simulink model "questao3Miguel"  (Simulink 8.7)
settings: Solver=ode45  StartTime=0.0  StopTime=40  MaxStep=0.01  RelTol=1e-3
values from neighbouring files (symbols this model uses):
  A = [0 1  0              0 ... (first row only)    [MatLab4p.m]    (also in MatLab5p.m = [     0        1       0        0; MatLab6p_solucao4.m = [     0        1       0        0; MatLab7p.m = [0 1; -5*sqrt(2) -1]; pplane8.m = [)
  Am = blkdiag(M,M)    [MatLab5p.m]    (also in MatLab6p_solucao4.m; questao2Miguel.m = blkdiag(M); questao2MiguelFinal.m = blkdiag(M))
  B = [0; 1/M; 0; -1/(M*L)]    [MatLab4p.m]    (also in MatLab5p.m = [ 0    0; MatLab6p_solucao4.m = [ 0    0; MatLab7p.m = [0 ; 10]; pplane8.m = real(A))
  Bm = blkdiag(N,N)    [MatLab5p.m]    (also in MatLab6p_solucao4.m; questao2Miguel.m = blkdiag(N); questao2MiguelFinal.m = blkdiag(N))
  C = [1 0 0 0]    [MatLab4p.m]    (also in MatLab5p.m = [1 0 0 0; MatLab6p_solucao4.m = [1 0 0 0; MatLab7p.m = [1 0]; pplane8.m = imag(A))
  Dsim = zeros(4,1)    [MatLab4p.m]    (also in MatLab5p.m = zeros(4,2); MatLab6p_solucao4.m = zeros(4,2); questao2Miguel.m; questao2MiguelFinal.m)
  g = 9.81    [MatLab4p.m]    (also in PenduloInvertidoNLinear.m; questao2Miguel.m; questao2MiguelFinal.m)
  K = place(A,B,[-3 -3.05 -3.1 -3.15])    [MatLab4p.m]    (also in MatLab5p.m = Ka(:,1:4); MatLab6p_solucao4.m = Ka(:,1:4); MatLab7p.m = place(A,B,[-4 -4.05]); pplane8.m = kk +2*(jj-1))
  Km = Ka(:,5:10)    [MatLab5p.m]    (also in MatLab6p_solucao4.m = Ka(:,5:12); MatLab7p.m = Ka(1,3); questao2Miguel.m = Ka(5); questao2MiguelFinal.m = Ka(5))
  L = (place(A',C',[-9 -9.05 -9.1 -9.15]))'    [MatLab4p.m]    (also in MatLab7p.m = [23 ; 113.9289]; PenduloInvertidoNLinear.m = 1; pplane8.m = length(t); questao2Miguel.m = 1)
  Lobs = H'    [MatLab6p_solucao4.m]    (also in questao2Miguel.m; questao2MiguelFinal.m)
  m = 0.5    [MatLab4p.m]    (also in PenduloInvertidoNLinear.m; questao2Miguel.m; questao2MiguelFinal.m)
  Mcar = 1    [questao2MiguelFinal.m]
  x0 = [0 0 pi/4 0]    [MatLab4p.m]    (also in MatLab5p.m = [1 0.5 1 0.1]; MatLab6p_solucao4.m = [0 0 0 0]; MatLab7p.m = [0 ; 0]; questao2Miguel.m = [0 0.01 0.3 0])
  x0obs = [0 0 0 0]    [MatLab4p.m]    (also in MatLab6p_solucao4.m; MatLab7p.m = [0 ; 0]; questao2Miguel.m; questao2MiguelFinal.m)
  xe = [0 0 pi 0]    [questao2MiguelFinal.m]
settings Model: Creator=hector  LastModifiedBy=Deinis-UFSC
settings DebuggingCC: UnderspecifiedInitializationDetection=Simplified  MergeDetectMultiDrivingBlocksExec=error  SolverPrmCheckMsg=warning
settings ConfigComp: CovSFcnEnable=off

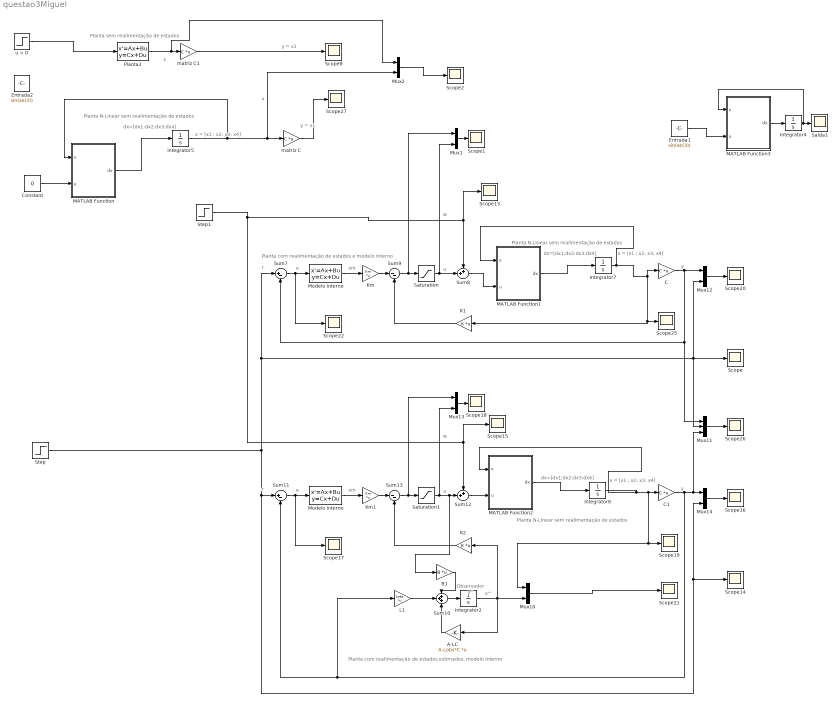
== system questao3Miguel ==
  note: Planta com realimentação de estados estimados, modelo interno
  note: Planta com realimentação de estados e modelo interno
  note: w
  note: u
  note: xm
  note: e
  note: r
  note: y
  note: w
  note: u
  note: xm
  note: e
  note: r
  note: y
  note: Observador
  note: x^
  note: x^
  note: Planta N-Linear sem realimentação de estados
  note: x
  note: y = x1
  note: dx=[dx1;dx2;dx3;dx4]
  note: x = [x1 ; x2; x3; x4]
  note: Planta N-Linear sem realimentação de estados
  note: dx=[dx1;dx2;dx3;dx4]
  note: x = [x1 ; x2; x3; x4]
  note: Planta N-Linear sem realimentação de estados
  note: dx=[dx1;dx2;dx3;dx4]
  note: x = [x1 ; x2; x3; x4]
  note: Planta sem realimentação de estados
  note: x
  note: y = x1
  A-LC : Gain  Gain=A-Lobs*C  Multiplication=Matrix(K*u)
  B1 : Gain  Gain=B  Multiplication=Matrix(K*u)
  C : Gain  Gain=C  Multiplication=Matrix(K*u)
  C1 : Gain  Gain=C  Multiplication=Matrix(K*u)
  Constant : Constant  Value=0
  Entrada1 : Constant  Value=sin(xe(3))
  Entrada2 : Constant  Value=sin(xe(3))
  Integrator2 : Integrator  InitialCondition=x0obs
  Integrator4 : Integrator  InitialCondition=xe
  Integrator5 : Integrator  InitialCondition=x0
  Integrator7 : Integrator  InitialCondition=x0
  Integrator8 : Integrator  InitialCondition=x0
  K1 : Gain  Gain=K  Multiplication=Matrix(K*u)
  K2 : Gain  Gain=K  Multiplication=Matrix(K*u)
  Km : Gain  Gain=Km  Multiplication=Matrix(K*u)
  Km1 : Gain  Gain=Km  Multiplication=Matrix(K*u)
  L1 : Gain  Gain=Lobs  Multiplication=Matrix(K*u)
  MATLAB Function : MATLAB Function  TreatAsAtomicUnit=on
  MATLAB Function1 : MATLAB Function  TreatAsAtomicUnit=on
  MATLAB Function2 : MATLAB Function  TreatAsAtomicUnit=on
  MATLAB Function3 : MATLAB Function  TreatAsAtomicUnit=on
  Modelo Interno : StateSpace  A=Am  B=Bm  D=0  X0=0
  Modelo interno : StateSpace  A=Am  B=Bm  D=0  X0=0
  Mux{1..2,10,12..14} (6 alike) : Mux  Inputs=2
  Mux11 : Mux  Inputs=3
  Planta2 : StateSpace  A=A  B=B  C=eye(4)  D=Dsim  X0=x0
  Saida1 : Scope
  Saturation : Saturate  UpperLimit=50  LowerLimit=-50
  Saturation1 : Saturate  UpperLimit=50  LowerLimit=-50
  Scope{,1..2,8,13..22,25..27} (17 alike) : Scope
  Step : Step  Time=5  SampleTime=0
  Step1 : Step  Time=15  After=0.5  SampleTime=0
  Sum10 : Sum  Inputs=+++
  Sum11 : Sum  Inputs=|+-
  Sum12 : Sum  Inputs=++|
  Sum13 : Sum  Inputs=|--
  Sum7 : Sum  Inputs=|+-
  Sum8 : Sum  Inputs=++|
  Sum9 : Sum  Inputs=|--
  matriz C : Gain  Gain=C  Multiplication=Matrix(K*u)
  matriz C1 : Gain  Gain=C  Multiplication=Matrix(K*u)
  "u = 0 " : Step  Time=0  After=0  SampleTime=0
  wires:
  Sum7/1 -> Modelo Interno/1, Scope22/1
  Mux12/1 -> Scope20/1
  Km/1 -> Sum9/1
  Modelo Interno/1 -> Km/1
  K1/1 -> Sum9/2
  Step/1 -> Sum7/1, Mux11/2, Scope/1, Mux12/2, Sum11/1, Scope14/1, Mux14/2
  Sum11/1 -> Modelo interno/1, Scope17/1
  Step1/1 -> Sum12/1, Scope15/1, Sum8/1, Scope13/1
  Mux14/1 -> Scope16/1
  Sum13/1 -> Mux13/1, Saturation1/1
  Km1/1 -> Sum13/1
  Modelo interno/1 -> Km1/1
  K2/1 -> Sum13/2
  Sum10/1 -> Integrator2/1
  L1/1 -> Sum10/2
  A-LC/1 -> Sum10/3
  B1/1 -> Sum10/1
  Mux10/1 -> Scope21/1
  Mux11/1 -> Scope26/1
  matriz C/1 -> Scope27/1
  Mux13/1 -> Scope18/1
  Constant/1 -> MATLAB Function/2(u)
  Sum8/1 -> MATLAB Function1/2(u)
  MATLAB Function1/1(dx) -> Integrator7/1
  Sum12/1 -> MATLAB Function2/2(u)
  MATLAB Function2/1(dx) -> Integrator8/1
  C1/1 -> L1/1, Sum11/2, Mux11/3, Mux14/1
  C/1 -> Mux12/1, Sum7/2, Mux11/1
  Integrator5/1 -> MATLAB Function/1(x), Mux2/2, matriz C/1
  Integrator7/1 -> MATLAB Function1/1(x), K1/1, Scope25/1, C/1
  Saturation1/1 -> Mux13/2, B1/1, Sum12/2
  Integrator2/1 -> A-LC/1, Mux10/2, K2/1
  Integrator8/1 -> Mux10/1, Scope19/1, C1/1, MATLAB Function2/1(x)
  MATLAB Function/1(dx) -> Integrator5/1
  Sum9/1 -> Mux1/1, Saturation/1
  Mux1/1 -> Scope1/1
  Saturation/1 -> Mux1/2, Sum8/2
  MATLAB Function3/1(dx) -> Integrator4/1
  Integrator4/1 -> MATLAB Function3/1(x), Saida1/1
  Entrada1/1 -> MATLAB Function3/2(u)
  "u = 0 "/1 -> Planta2/1
  matriz C1/1 -> Scope8/1
  Planta2/1 -> Mux2/1, matriz C1/1
  Mux2/1 -> Scope2/1

== matlab function MATLAB Function1 ==
  data: x input double; u input double; dx output double; m parameter double; Mcar parameter double; L parameter double; g parameter double
function dx = fcn(x,u,m, Mcar, L, g)
%#codegen

% dx1 = x(2);
% dx2 = u - (m*g*cos(x(3))*sin(x(3))+m*L*x(4)^2*sin(x(3)))/(Mcar+m - m*cos(x(3))^2);
% dx3 = x(4);
% dx4 = (u*cos(x(3))+m*L*x(4)^2*cos(x(3))*sin(x(3))-(Mcar+m)*g*sin(x(3)))/(m*L*cos(x(3))^2 - L*(Mcar+m));

dx1 = x(2);
dx2 = (m*L*x(4)^2*sin(x(3))-m*g*sin(x(3))*cos(x(3)) + u)/((Mcar+m*sin(x(3))^2)*L);
dx3 = x(4);
dx4 = ((Mcar+m)*g*sin(x(3)) + m*L*x(4)^2*sin(x(3))*cos(x(3)) - u*cos(x(3)))/((Mcar+m*sin(x(3))^2)*L);

dx = [dx1 ; dx2 ; dx3 ; dx4];

== matlab function MATLAB Function ==
  data: x input double; u input double; dx output double; m parameter double; Mcar parameter double; L parameter double; g parameter double
function dx = fcn(x,u,m, Mcar, L, g)
%#codegen

% dx1 = x(2);
% dx2 = u - (m*g*cos(x(3))*sin(x(3))+m*L*x(4)^2*sin(x(3)))/(Mcar+m - m*cos(x(3))^2);
% dx3 = x(4);
% dx4 = (u*cos(x(3))+m*L*x(4)^2*cos(x(3))*sin(x(3))-(Mcar+m)*g*sin(x(3)))/(m*L*cos(x(3))^2 - L*(Mcar+m));

dx1 = x(2);
dx2 = (m*L*x(4)^2*sin(x(3))-m*g*sin(x(3))*cos(x(3)) + u)/((Mcar+m*sin(x(3))^2)*L);
dx3 = x(4);
dx4 = ((Mcar+m)*g*sin(x(3)) + m*L*x(4)^2*sin(x(3))*cos(x(3)) - u*cos(x(3)))/((Mcar+m*sin(x(3))^2)*L);

dx = [dx1 ; dx2 ; dx3 ; dx4];

== matlab function MATLAB Function2 ==
  data: x input double; u input double; dx output double; m parameter double; Mcar parameter double; L parameter double; g parameter double
function dx = fcn(x,u,m, Mcar, L, g)
%Miguel 

% dx1 = x(2);
% dx2 = u - (m*g*cos(x(3))*sin(x(3))+m*L*x(4)^2*sin(x(3)))/(Mcar+m - m*cos(x(3))^2);
% dx3 = x(4);
% dx4 = (u*cos(x(3))+m*L*x(4)^2*cos(x(3))*sin(x(3))-(Mcar+m)*g*sin(x(3)))/(m*L*cos(x(3))^2 - L*(Mcar+m));

dx1 = x(2);
dx2 = (m*L*x(4)^2*sin(x(3))-m*g*sin(x(3))*cos(x(3)) + u)/((Mcar+m*sin(x(3))^2)*L);
dx3 = x(4);
dx4 = ((Mcar+m)*g*sin(x(3)) + m*L*x(4)^2*sin(x(3))*cos(x(3)) - u*cos(x(3)))/((Mcar+m*sin(x(3))^2)*L);


dx = [dx1 ; dx2 ; dx3 ; dx4];

== matlab function MATLAB Function3 ==
  data: x input double; u input double; dx output double; m parameter double; Mcar parameter double; L parameter double; g parameter double
function dx = fcn(x,u,m, Mcar, L, g)
%#codegen

% dx1 = x(2);
% dx2 = u - (m*g*cos(x(3))*sin(x(3))+m*L*x(4)^2*sin(x(3)))/(Mcar+m - m*cos(x(3))^2);
% dx3 = x(4);
% dx4 = (u*cos(x(3))+m*L*x(4)^2*cos(x(3))*sin(x(3))-(Mcar+m)*g*sin(x(3)))/(m*L*cos(x(3))^2 - L*(Mcar+m));

dx1 = x(2);
dx2 = (m*L*x(4)^2*sin(x(3))-m*g*sin(x(3))*cos(x(3)) + u)/((Mcar+m*sin(x(3))^2)*L);
dx3 = x(4);
dx4 = ((Mcar+m)*g*sin(x(3)) + m*L*x(4)^2*sin(x(3))*cos(x(3)) - u*cos(x(3)))/((Mcar+m*sin(x(3))^2)*L);

dx = [dx1 ; dx2 ; dx3 ; dx4];
